simulink model "simulacion_loopshaping"  (R2022b)
settings: Solver=VariableStepAuto  StartTime=0.0  StopTime=20  RelTol=1e-3
values from neighbouring files (symbols this model uses):
  beta = gamma*2*I    (= 0.0001265)    [parametros.m]
  db = 4.2/100    (= 0.042)    [parametros.m]
  dc = 5/100    (= 0.05)    [parametros.m]
  dm = 13.1/100    (= 0.131)    [parametros.m]
  g = 9.81    [parametros.m]
  I = 1.1e-4    (= 0.00011)    [parametros.m]
  mb = 7.38/1000    (= 0.00738)    [parametros.m]
  mc = 2.07/1000    (= 0.00207)    [parametros.m]
  mm = (3.2+1.28)/1000    (= 0.00448)    [parametros.m]
undefined symbols (not defined in the file or in its folder): K_ls, TF, tf_polo_real
settings Model: Creator=danie  LastModifiedBy=danie

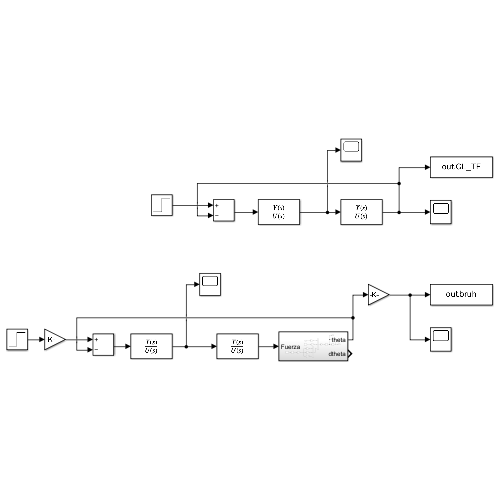
[thumbnail: Simulink's stored preview of the top-level diagram]
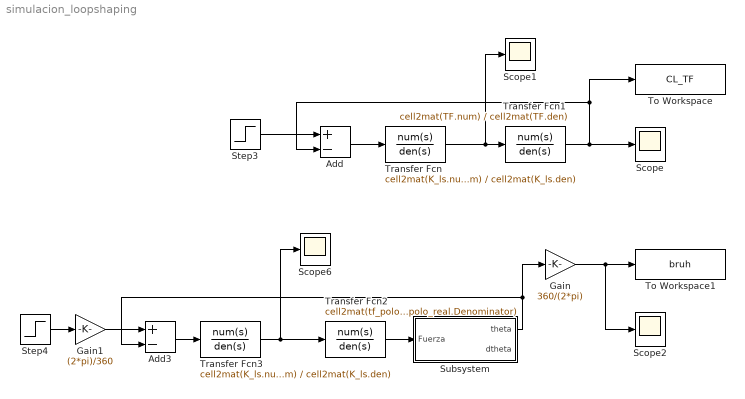
== system simulacion_loopshaping ==
  Add : Sum  Inputs=+-
  Add3 : Sum  Inputs=+-
  Gain : Gain  Gain=360/(2*pi)
  Gain1 : Gain  Gain=(2*pi)/360
  Scope{,1..2,6} (4 alike) : Scope
  Step3 : Step  After=150  SampleTime=0
  Step4 : Step  After=90  SampleTime=0
  Subsystem : Subsystem
  To Workspace : ToWorkspace  VariableName=CL_TF  SaveFormat=Timeseries  SampleTime=-1
  To Workspace1 : ToWorkspace  VariableName=bruh  SaveFormat=Timeseries  SampleTime=-1
  Transfer Fcn : TransferFcn  Numerator=cell2mat(K_ls.num)  Denominator=cell2mat(K_ls.den)
  Transfer Fcn1 : TransferFcn  Numerator=cell2mat(TF.num)  Denominator=cell2mat(TF.den)
  Transfer Fcn2 : TransferFcn  Numerator=cell2mat(tf_polo_real.Numerator)  Denominator=cell2mat(tf_polo_real.Denominator)
  Transfer Fcn3 : TransferFcn  Numerator=cell2mat(K_ls.num)  Denominator=cell2mat(K_ls.den)
  wires:
  Transfer Fcn1/1 -> To Workspace/1, Add/2, Scope/1
  Add/1 -> Transfer Fcn/1
  Transfer Fcn/1 -> Scope1/1, Transfer Fcn1/1
  Gain/1 -> To Workspace1/1, Scope2/1
  Transfer Fcn2/1 -> Subsystem/1(Fuerza)
  Step3/1 -> Add/1
  Step4/1 -> Gain1/1
  Add3/1 -> Transfer Fcn3/1
  Subsystem/1(theta) -> Add3/2, Gain/1
  Gain1/1 -> Add3/1
  Transfer Fcn3/1 -> Transfer Fcn2/1, Scope6/1

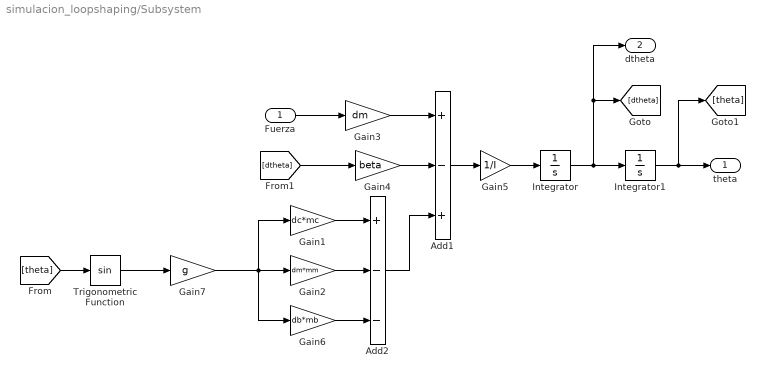
== system simulacion_loopshaping/Subsystem ==
  Fuerza : Inport
  Add1 : Sum  Inputs=+-+
  Add2 : Sum  Inputs=+--
  Gain1 : Gain  Gain=dc*mc
  Gain2 : Gain  Gain=dm*mm
  Gain3 : Gain  Gain=dm
  Gain4 : Gain  Gain=beta
  Gain5 : Gain  Gain=1/I
  Gain6 : Gain  Gain=db*mb
  Gain7 : Gain  Gain=g
  Integrator : Integrator
  Integrator1 : Integrator
  Trigonometric Function : Trigonometry
  theta : Outport
  dtheta : Outport  Port=2
  wires:
  Gain4/1 -> Add1/2
  Gain5/1 -> Integrator/1
  Add1/1 -> Gain5/1
  [dtheta] -> Gain4/1
  [theta] -> Trigonometric Function/1
  Integrator/1 -> dtheta/1, [dtheta], Integrator1/1
  Integrator1/1 -> [theta], theta/1
  Fuerza/1 -> Gain3/1
  Gain1/1 -> Add2/1
  Gain2/1 -> Add2/2
  Gain6/1 -> Add2/3
  Add2/1 -> Add1/3
  Trigonometric Function/1 -> Gain7/1
  Gain3/1 -> Add1/1
  Gain7/1 -> Gain6/1, Gain2/1, Gain1/1
